simulink model "FromEntradatoGananciaToworkspace"  (R2018a)
settings: Solver=ode4  StartTime=0.0  StopTime=10.0  FixedStep=0.05  RelTol=1e-3
settings Model: Creator=adtenla  LastModifiedBy=adtenla

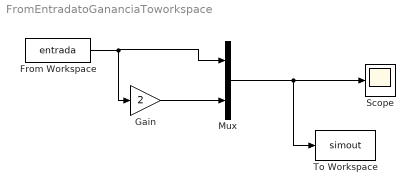
== system FromEntradatoGananciaToworkspace ==
  From Workspace : FromWorkspace  VariableName=entrada  SampleTime=0
  Gain : Gain  Gain=2
  Mux : Mux  Inputs=2
  Scope : Scope
  To Workspace : ToWorkspace  VariableName=simout  SampleTime=-1
  wires:
  From Workspace/1 -> Mux/1, Gain/1
  Gain/1 -> Mux/2
  Mux/1 -> To Workspace/1, Scope/1
